simulink model "step2"  (R2021b)
settings: Solver=VariableStepAuto  StartTime=0.0  StopTime=10.0  RelTol=1e-3
settings Model: Creator=just cookie file  LastModifiedBy=just cookie file

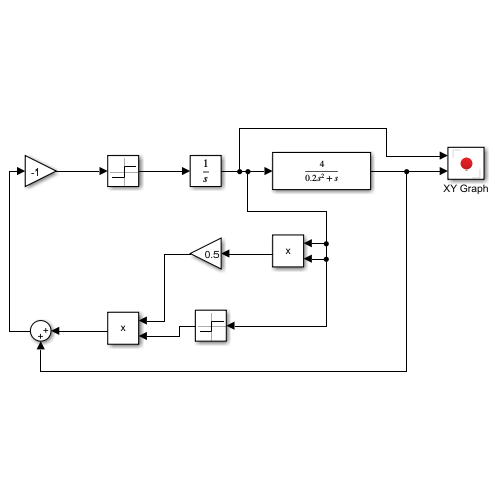
[thumbnail: Simulink's stored preview of the top-level diagram]
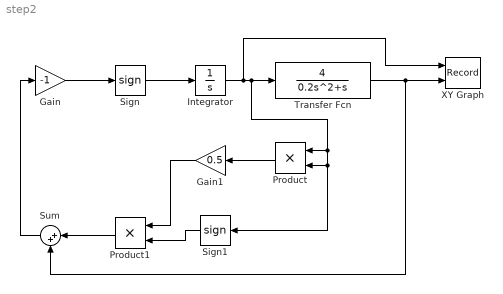
== system step2 ==
  Gain : Gain  Gain=-1
  Gain1 : Gain  Gain=0.5
  Integrator : Integrator  InitialCondition=1
  Product : Product
  Product1 : Product
  Sign : Signum  ZeroCross=off
  Sign1 : Signum  ZeroCross=off
  Sum : Sum  Inputs=|++
  Transfer Fcn : TransferFcn  Numerator=[4]  Denominator=[0.2 1 0]
  XY Graph : Record  FileSettingsInternal="{\"entries\":[{\"content\":{\"excelSettings\":{\"content\":{},\"type\":\"Streamout.ExcelSettings\"}},\"type\":\"Streamout.FileSettingStorage\",\"uuid\":\"c8f97f76-8aca-4c8a-98d0-985f608419e3\"}],\"packageUris\":[\"http://schema.mathworks.com/mf0/streamout_blocks/R2020a\"],\"version\":\"1.0\"}"  Layout=[1 1]  SignalsInternal="{\"entries\":[{\"content\":{\"signals\":[{\"content\":{\"blockPath\":[\"untitled/XY Graph\"],\"channel\":[],\"dimensions\":[1],\"domain\":\"untitled/XY Graph\",\"lineColor\":\"#a2142f\",\"plots\":[1],\"port\":1,\"sid\":[\"\"],\"signalID\":245,\"signalName\":\"Integrator\"},\"type\":\"RecordBlkView.Signal\",\"uuid\":\"fd21f589-4316-40f1-8140-661978f37138\"},{\"content\":{\"blockPath\":[\"untitled/XY Graph\"],\"channel\":[],\"dimensions\":[1],\"domain\":\"untitled/XY Graph\",\"lineColor\":\"#139fff\",\"plots\":[1],\"port\":2,\"sid\":[\"\"],\"signalID\":249,\"signalName\":\"Transfer Fcn\"},\"type\":\"RecordBlkView.Signal\",\"uuid\":\"5bceab78-7410-485a-819f-20b435b3a4e8\"}]},\"type\":\"RecordBlkView.InputSignals\",\"uuid\":\"2a838917-64ee-456c-8dff-870ef70ac825\"}],\"packageUris\":[\"http://schema.mathworks.com/mf0/streamout_blocks/R2020a\"],\"version\":\"1.0\"}"  VisualizationBindings="{\"xyplotplugin\":{\"info\":[{\"series\":[{\"bindingParametersList\":[{\"parameter\":\"X-Axis\",\"signalID\":245,\"signalName\":\"Integrator\"},{\"parameter\":\"Y-Axis\",\"signalID\":249,\"signalName\":\"Transfer Fcn\"}],\"seriesID\":39876}],\"subplotID\":1}]}}"  CompatibilityTag=XY
  wires:
  Sum/1 -> Gain/1
  Gain/1 -> Sign/1
  Sign/1 -> Integrator/1
  Integrator/1 -> Transfer Fcn/1, Product/2, Sign1/1, Product/1, XY Graph/1
  Transfer Fcn/1 -> Sum/2, XY Graph/2
  Product/1 -> Gain1/1
  Product1/1 -> Sum/1
  Sign1/1 -> Product1/2
  Gain1/1 -> Product1/1
